simulink model "sys"  (R2025b)
settings: Solver=FixedStepDiscrete  StartTime=0.0  StopTime=simin.Time.data(end)  FixedStep=0.001  RelTol=1e-3
model workspace (MAT data in the model file):
  Fz_stat_FL = Simulink.Parameter
  Fz_stat_FL.Value = 3921.3656
  Fz_stat_FL.Complexity = 'real'
  Fz_stat_FL.Dimensions = [1 1]
  Fz_stat_FL.DataType = 'double'
  Fz_stat_FL.DocUnits = 'N'
  Fz_stat_FR = Simulink.Parameter
  Fz_stat_FR.Value = 3921.3656
  Fz_stat_FR.Complexity = 'real'
  Fz_stat_FR.Dimensions = [1 1]
  Fz_stat_FR.DataType = 'double'
  Fz_stat_FR.DocUnits = 'N'
  Fz_stat_RL = Simulink.Parameter
  Fz_stat_RL.Value = 3922.1269
  Fz_stat_RL.Complexity = 'real'
  Fz_stat_RL.Dimensions = [1 1]
  Fz_stat_RL.DataType = 'double'
  Fz_stat_RL.DocUnits = 'N'
  Fz_stat_RR = Simulink.Parameter
  Fz_stat_RR.Value = 3922.1267
  Fz_stat_RR.Complexity = 'real'
  Fz_stat_RR.Dimensions = [1 1]
  Fz_stat_RR.DataType = 'double'
  Fz_stat_RR.DocUnits = 'N'
  cog_height = Simulink.Parameter
  cog_height.Value = 0.604
  cog_height.Complexity = 'real'
  cog_height.Dimensions = [1 1]
  cog_height.DataType = 'double'
  cog_height.DocUnits = 'm'
  g = Simulink.Parameter
  g.Value = 9.806
  g.Complexity = 'real'
  g.Dimensions = [1 1]
  g.DataType = 'double'
  g.DocUnits = 'm/s^2'
  lF = Simulink.Parameter
  lF.Value = 1.466
  lF.Complexity = 'real'
  lF.Dimensions = [1 1]
  lF.DataType = 'double'
  lF.DocUnits = 'm'
  lR = Simulink.Parameter
  lR.Value = 1.509
  lR.Complexity = 'real'
  lR.Dimensions = [1 1]
  lR.DataType = 'double'
  lR.DocUnits = 'm'
  pitchAngle = Simulink.Parameter
  pitchAngle.Value = [0.00443372596055 0.00472012698538 0.00500652801021 0.00529292903504 0.00557933005986 0.00586573108469 0.00615213210952 0.00643853313435 0.00672493415917 0.007011335184 0.00729773620883 0.00758413723366 ... (200 elements, 200x1)]
  pitchAngle.Complexity = 'real'
  pitchAngle.Dimensions = [200 1]
  pitchAngle.DataType = 'double'
  pitchAngle.DocUnits = 'rad'
  pitchStiffness = Simulink.Parameter
  pitchStiffness.Value = [286621.759635 286644.842257 286407.773968 286374.136656 286600.567598 286901.705993 287109.32323 287190.659823 287245.018359 287344.728913 287488.533524 287631.863692 ... (200 elements, 200x1)]
  pitchStiffness.Complexity = 'real'
  pitchStiffness.Dimensions = [200 1]
  pitchStiffness.DataType = 'double'
  pitchStiffness.DocUnits = 'N*m/rad'
  pitch_inertia = Simulink.Parameter
  pitch_inertia.Value = 2180.5
  pitch_inertia.Complexity = 'real'
  pitch_inertia.Dimensions = [1 1]
  pitch_inertia.DataType = 'double'
  pitch_inertia.DocUnits = 'kg * m^2'
  pitching_coefficient = Simulink.Parameter
  pitching_coefficient.Value = -0.002
  pitching_coefficient.Complexity = 'real'
  pitching_coefficient.Dimensions = [1 1]
  pitching_coefficient.DataType = 'double'
  pitching_coefficient.DocUnits = '1'
  r = 0.9402
  rdyn = Simulink.Parameter
  rdyn.Value = 0.309
  rdyn.Complexity = 'real'
  rdyn.Dimensions = [1 1]
  rdyn.DataType = 'double'
  rdyn.DocUnits = 'm'
  reference_area = Simulink.Parameter
  reference_area.Value = 2.4
  reference_area.Complexity = 'real'
  reference_area.Dimensions = [1 1]
  reference_area.DataType = 'double'
  reference_area.DocUnits = 'kg / m^3'
  rho = Simulink.Parameter
  rho.Value = 1.2
  rho.Complexity = 'real'
  rho.Dimensions = [1 1]
  rho.DataType = 'double'
  rho.DocUnits = 'm^2'
  rollStiffness_F = Simulink.Parameter
  rollStiffness_F.Value = -66168.4036
  rollStiffness_F.Complexity = 'real'
  rollStiffness_F.Dimensions = [1 1]
  rollStiffness_F.DataType = 'double'
  rollStiffness_F.DocUnits = 'N*m/rad'
  rollStiffness_R = Simulink.Parameter
  rollStiffness_R.Value = -79058.3706
  rollStiffness_R.Complexity = 'real'
  rollStiffness_R.Dimensions = [1 1]
  rollStiffness_R.DataType = 'double'
  rollStiffness_R.DocUnits = 'N*m/rad'
  sprung_mass = Simulink.Parameter
  sprung_mass.Value = 1373.3
  sprung_mass.Complexity = 'real'
  sprung_mass.Dimensions = [1 1]
  sprung_mass.DataType = 'double'
  sprung_mass.DocUnits = 'kg'
  total_pitchDamping = Simulink.Parameter
  total_pitchDamping.Value = 22000
  total_pitchDamping.Complexity = 'real'
  total_pitchDamping.Dimensions = [1 1]
  total_pitchDamping.DataType = 'double'
  total_pitchDamping.DocUnits = 'N*m/rad'
  total_pitchStiffness = Simulink.Parameter
  total_pitchStiffness.Value = 291158.1055
  total_pitchStiffness.Complexity = 'real'
  total_pitchStiffness.Dimensions = [1 1]
  total_pitchStiffness.DataType = 'double'
  total_pitchStiffness.DocUnits = 'N*m/rad'
  total_rollStiffness = Simulink.Parameter
  total_rollStiffness.Value = 138201.9734
  total_rollStiffness.Complexity = 'real'
  total_rollStiffness.Dimensions = [1 1]
  total_rollStiffness.DataType = 'double'
  total_rollStiffness.DocUnits = 'N*m/rad'
  total_rollStifness = Simulink.Parameter
  total_rollStifness.Value = 138201.9734
  total_rollStifness.Complexity = 'real'
  total_rollStifness.Dimensions = [1 1]
  total_rollStifness.DataType = 'double'
  total_rollStifness.DocUnits = 'Nm/rad'
  trackwidth_F = Simulink.Parameter
  trackwidth_F.Value = 1.6
  trackwidth_F.Complexity = 'real'
  trackwidth_F.Dimensions = [1 1]
  trackwidth_F.DataType = 'double'
  trackwidth_F.DocUnits = 'm'
  trackwidth_R = Simulink.Parameter
  trackwidth_R.Value = 1.614
  trackwidth_R.Complexity = 'real'
  trackwidth_R.Dimensions = [1 1]
  trackwidth_R.DataType = 'double'
  trackwidth_R.DocUnits = 'm'
  unsprung_mass = Simulink.Parameter
  unsprung_mass.Value = 226.704
  unsprung_mass.Complexity = 'real'
  unsprung_mass.Dimensions = [1 1]
  unsprung_mass.DataType = 'double'
  unsprung_mass.DocUnits = 'kg'
  wheelbase = Simulink.Parameter
  wheelbase.Value = 2.975
  wheelbase.Complexity = 'real'
  wheelbase.Dimensions = [1 1]
  wheelbase.DataType = 'double'
  wheelbase.DocUnits = 'm'
undefined symbols (not defined in the file): DiscIntNeverNeededParam
settings Model: Creator=I012488  LastModifiedBy=marcelkaminski
settings DebuggingCC: UnconnectedInputMsg=warning  UnconnectedOutputMsg=warning  UnconnectedLineMsg=warning
settings ModelReferenceCC: EnableRefExpFcnMdlSchedulingChecks=on
settings RTWCC: GPUComputeCapability=3.5  DLArmComputeVersion=19.05

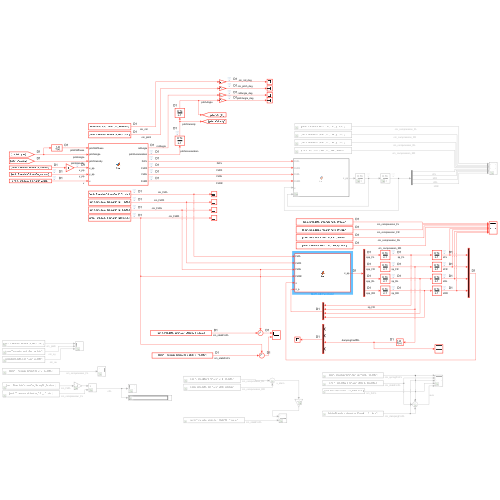
[thumbnail: Simulink's stored preview of the top-level diagram]
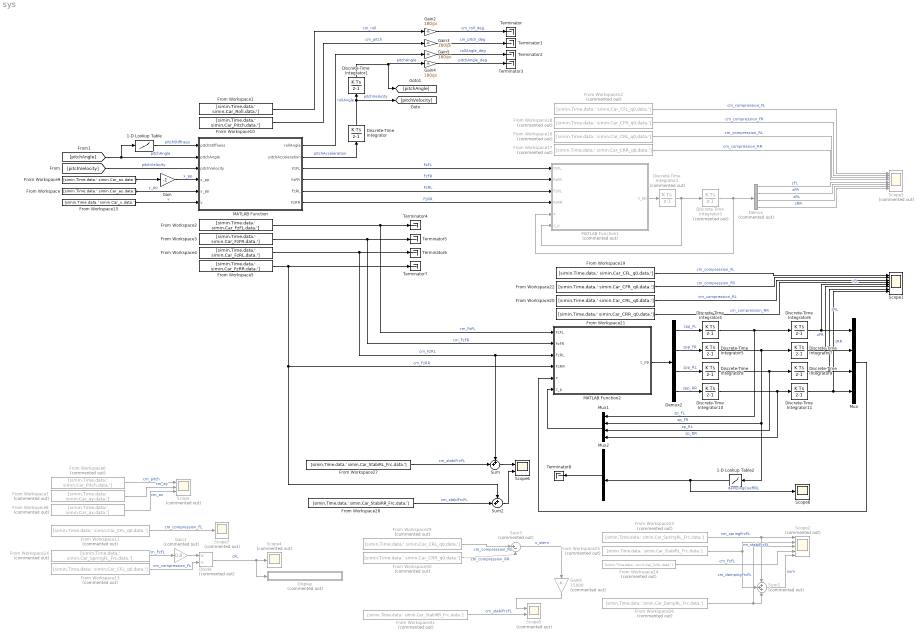
== system sys ==
  1-D Lookup Table : Lookup_n-D  NumberOfTableDimensions=1  BreakpointsForDimension1=pitchAngle  Table=pitchStiffness  InternalRulePriority=Speed  RndMeth=Simplest
  1-D Lookup Table2 : Lookup_n-D  NumberOfTableDimensions=1  BreakpointsForDimension1=[-1 -0.1 0 0.1 1]  Table="[2055.90  31.359 0 18.453 756.31]"  InternalRulePriority=Speed  RndMeth=Simplest
  Demux : Demux  Commented=on
  Demux2 : Demux
  Discrete-Time Integrator{,4..8,10..11} (8 alike) : DiscreteIntegrator  SampleTime=-1  ICPrevOutput=DiscIntNeverNeededParam  ICPrevScaledInput=DiscIntNeverNeededParam
  Discrete-Time Integrator1 : DiscreteIntegrator  InitialCondition=-0.001  SampleTime=-1  ICPrevOutput=DiscIntNeverNeededParam  ICPrevScaledInput=DiscIntNeverNeededParam
  Discrete-Time Integrator2 : DiscreteIntegrator  Commented=on  SampleTime=-1  ICPrevOutput=DiscIntNeverNeededParam  ICPrevScaledInput=DiscIntNeverNeededParam
  Discrete-Time Integrator3 : DiscreteIntegrator  Commented=on  SampleTime=-1  ICPrevOutput=DiscIntNeverNeededParam  ICPrevScaledInput=DiscIntNeverNeededParam
  Discrete-Time Integrator9 : DiscreteIntegrator  InitialCondition=-0.0007  SampleTime=-1  ICPrevOutput=DiscIntNeverNeededParam  ICPrevScaledInput=DiscIntNeverNeededParam
  Display : Display  Commented=on
      settings: Format=long_e
  Divide : Product  Commented=on  Inputs=*/
  From Workspace : FromWorkspace  VariableName=[simin.Time.data.' simin.Car_ay.data.']  SampleTime=0.01
  From Workspace1 : FromWorkspace  VariableName=[simin.Time.data.' simin.Car_Roll.data.']  SampleTime=0.01
  From Workspace10 : FromWorkspace  VariableName=[simin.Time.data.' simin.Car_Pitch.data.']  SampleTime=0.01
  From Workspace11 : FromWorkspace  Commented=on  VariableName=[simin.Time.data.' simin.Car_CFL_q0.data.']
  From Workspace12 : FromWorkspace  Commented=on  VariableName=[simin.Time.data.' simin.Car_CFL_q0.data.']  SampleTime=0.01
  From Workspace13 : FromWorkspace  Commented=on  VariableName=[simin.Time.data.' simin.Car_CFL_q0.data.']
  From Workspace14 : FromWorkspace  Commented=on  VariableName=[simin.Time.data.' simin.Car_SpringFL_Frc.data.']
  From Workspace15 : FromWorkspace  VariableName=[simin.Time.data.' simin.Car_v.data.']  SampleTime=0.01
  From Workspace16 : FromWorkspace  Commented=on  VariableName=[simin.Time.data.' simin.Car_CRL_q0.data.']  SampleTime=0.01
  From Workspace17 : FromWorkspace  Commented=on  VariableName=[simin.Time.data.' simin.Car_CRR_q0.data.']  SampleTime=0.01
  From Workspace18 : FromWorkspace  Commented=on  VariableName=[simin.Time.data.' simin.Car_CFR_q0.data.']  SampleTime=0.01
  From Workspace19 : FromWorkspace  VariableName=[simin.Time.data.' simin.Car_CFL_q0.data.']  SampleTime=0.01
  From Workspace2 : FromWorkspace  VariableName=[simin.Time.data.' simin.Car_FzFL.data.']  SampleTime=0.01
  From Workspace20 : FromWorkspace  VariableName=[simin.Time.data.' simin.Car_CRL_q0.data.']  SampleTime=0.01
  From Workspace21 : FromWorkspace  VariableName=[simin.Time.data.' simin.Car_CRR_q0.data.']  SampleTime=0.01
  From Workspace22 : FromWorkspace  VariableName=[simin.Time.data.' simin.Car_CFR_q0.data.']  SampleTime=0.01
  From Workspace23 : FromWorkspace  Commented=on  VariableName=[simin.Time.data.' simin.Car_SpringRL_Frc.data.']  SampleTime=0.01
  From Workspace24 : FromWorkspace  Commented=on  VariableName=[simin.Time.data.' simin.Car_FzRL.data.']  SampleTime=0.01
  From Workspace25 : FromWorkspace  Commented=on  VariableName=[simin.Time.data.' simin.Car_StabiRL_Frc.data.']  SampleTime=0.01
  From Workspace26 : FromWorkspace  Commented=on  VariableName=[simin.Time.data.' simin.Car_DampRL_Frc.data.']  SampleTime=0.01
  From Workspace27 : FromWorkspace  VariableName=[simin.Time.data.' simin.Car_StabiRL_Frc.data.']  SampleTime=0.01
  From Workspace28 : FromWorkspace  VariableName=[simin.Time.data.' simin.Car_StabiRR_Frc.data.']  SampleTime=0.01
  From Workspace29 : FromWorkspace  Commented=on  VariableName=[simin.Time.data.' simin.Car_CRL_q0.data.']  SampleTime=0.01
  From Workspace3 : FromWorkspace  VariableName=[simin.Time.data.' simin.Car_FzFR.data.']  SampleTime=0.01
  From Workspace30 : FromWorkspace  Commented=on  VariableName=[simin.Time.data.' simin.Car_CRR_q0.data.']  SampleTime=0.01
  From Workspace31 : FromWorkspace  Commented=on  VariableName=[simin.Time.data.' simin.Car_StabiRR_Frc.data.']  SampleTime=0.01
  From Workspace4 : FromWorkspace  VariableName=[simin.Time.data.' simin.Car_FzRL.data.']  SampleTime=0.01
  From Workspace5 : FromWorkspace  VariableName=[simin.Time.data.' simin.Car_FzRR.data.']  SampleTime=0.01
  From Workspace6 : FromWorkspace  Commented=on  VariableName=[simin.Time.data.' simin.Car_Pitch.data.']
  From Workspace7 : FromWorkspace  Commented=on  VariableName=[simin.Time.data.' simin.Car_ay.data.']
  From Workspace8 : FromWorkspace  Commented=on  VariableName=[simin.Time.data.' simin.Car_ax.data.']
  From Workspace9 : FromWorkspace  VariableName=[simin.Time.data.' simin.Car_ax.data.']  SampleTime=0.01
  Gain : Gain  Gain=-1
  Gain1 : Gain  Commented=on  Gain=0.8
  Gain{2..5} (4 alike) : Gain  Gain=180/pi
  Gain6 : Gain  Commented=on  Gain=15000
  MATLAB Function : MATLAB Function  TreatAsAtomicUnit=on
  MATLAB Function1 : MATLAB Function  Commented=on  TreatAsAtomicUnit=on
  MATLAB Function2 : MATLAB Function  TreatAsAtomicUnit=on
  Mux : Mux
  Mux1 : Mux
  Mux2 : Mux
  Scope : Scope  Commented=on  NumInputPorts=3
      settings: ActiveDisplayYMinimum=-0.00699  ActiveDisplayYMaximum=0.02856  DataLoggingVariableName=ScopeData2
  Scope1 : Scope  NumInputPorts=8
      settings: ActiveDisplayYMinimum=-0.057258109748267769  ActiveDisplayYMaximum=0.059973873910534263
  Scope2 : Scope  Commented=on  NumInputPorts=5
      settings: ActiveDisplayYMinimum=-519.06918168067921  ActiveDisplayYMaximum=4484.9822962284088  DataLoggingVariableName=ScopeData4
  Scope3 : Scope  Commented=on  NumInputPorts=8
      settings: ActiveDisplayYMinimum=-0.094623233695607184  ActiveDisplayYMaximum=0.027480534772711229  DataLoggingVariableName=ScopeData2
  Scope4 : Scope  Commented=on
      settings: ActiveDisplayYMinimum=-6.64271465116E+8  ActiveDisplayYMaximum=3.41636027705721E+9  DataLoggingVariableName=ScopeData3
  Scope5 : Scope  Commented=on  NumInputPorts=2
      settings: ActiveDisplayYMinimum=-982.79968407035688  ActiveDisplayYMaximum=303.75455820689251  DataLoggingVariableName=ScopeData5
  Scope6 : Scope  NumInputPorts=2
      settings: ActiveDisplayYMinimum=-1  ActiveDisplayYMaximum=1  DataLoggingVariableName=ScopeData6
  Scope7 : Scope  Commented=on
      settings: ActiveDisplayYMinimum=-0.02942  ActiveDisplayYMaximum=0.01092
  Scope8 : Scope
      settings: ActiveDisplayYMinimum=-0.83271159099636516  ActiveDisplayYMaximum=7.4944043189672884  DataLoggingVariableName=ScopeData7
  Sum : Sum  Inputs=++|
  Sum1 : Sum  Commented=on  Inputs=+++
  Sum2 : Sum  Inputs=++|
  Sum3 : Sum  Commented=on  Inputs=|+-
  Terminator{,1..8} (9 alike) : Terminator
  wires:
  MATLAB Function/3(FzFL) -> MATLAB Function1/1(FzFL)  "FzFL"
  From Workspace/1 -> MATLAB Function/5(y_pp)  "y_pp"
  MATLAB Function/1(rollAngle) -> Gain5/1  "rollAngle"
  From Workspace1/1 -> Gain2/1  "cm_roll"
  From Workspace2/1 -> MATLAB Function2/1(FzFL), Terminator4/1  "cm_FzFL"
  MATLAB Function/4(FzFR) -> MATLAB Function1/2(FzFR)  "FzFR"
  MATLAB Function/5(FzRL) -> MATLAB Function1/3(FzRL)  "FzRL"
  MATLAB Function/6(FzRR) -> MATLAB Function1/4(FzRR)  "FzRR"
  From Workspace3/1 -> MATLAB Function2/2(FzFR), Terminator5/1  "cm_FzFR"
  From Workspace4/1 -> Sum/1, MATLAB Function2/3(FzRL), Terminator6/1  "cm_FzRL"
  From Workspace5/1 -> Terminator7/1, Sum2/1, MATLAB Function2/4(FzRR)  "cm_FzRR"
  From Workspace6/1 -> Scope/1  "cm_pitch"
  From Workspace7/1 -> Scope/2  "cm_ay"
  From Workspace8/1 -> Scope/3  "cm_ax"
  From Workspace9/1 -> Gain/1
  MATLAB Function1/1(z_pp) -> Discrete-Time Integrator2/1
  MATLAB Function/2(pitchAcceleration) -> Discrete-Time Integrator/1  "pitchAcceleration"
  From Workspace10/1 -> Gain3/1  "cm_pitch"
  Gain/1 -> MATLAB Function/4(x_pp)  "x_pp"
  From Workspace11/1 -> Scope7/1  "cm_compression_FL"
  From Workspace12/1 -> Scope3/1  "cm_compression_FL"
  Discrete-Time Integrator2/1 -> MATLAB Function1/6(z_p), Discrete-Time Integrator3/1
  Discrete-Time Integrator3/1 -> MATLAB Function1/5(z), Demux/1
  From Workspace14/1 -> Gain1/1  "cm_FzFL"
  From Workspace13/1 -> Divide/2  "cm_compression_FL"
  Divide/1 -> Display/1, Scope4/1  "cFL"
  Gain1/1 -> Divide/1
  Discrete-Time Integrator/1 -> [pitchVelocity], Discrete-Time Integrator1/1  "pitchVelocity"
  Discrete-Time Integrator1/1 -> Gain4/1, [pitchAngle]  "pitchAngle"
  [pitchVelocity] -> MATLAB Function/3(pitchVelocity)  "pitchVelocity"
  [pitchAngle] -> 1-D Lookup Table/1, MATLAB Function/2(pitchAngle)  "pitchAngle"
  From Workspace15/1 -> MATLAB Function/6(v)  "v"
  1-D Lookup Table/1 -> MATLAB Function/1(pitchStiffness)  "pitchStiffness"
  Gain2/1 -> Terminator/1  "cm_roll_deg"
  Gain3/1 -> Terminator1/1  "cm_pitch_deg"
  Gain4/1 -> Terminator3/1  "pitchAngle_deg"
  Gain5/1 -> Terminator2/1  "rollAngle_deg"
  From Workspace18/1 -> Scope3/2  "cm_compression_FR"
  From Workspace16/1 -> Scope3/3  "cm_compression_RL"
  From Workspace17/1 -> Scope3/4  "cm_compression_RR"
  Demux/1 -> Scope3/5  "zFL"
  Demux/2 -> Scope3/6  "zFR"
  Demux/3 -> Scope3/7  "zRL"
  Demux/4 -> Scope3/8  "zRR"
  From Workspace22/1 -> Scope1/2  "cm_compression_FR"
  From Workspace21/1 -> Scope1/4  "cm_compression_RR"
  From Workspace20/1 -> Scope1/3  "cm_compression_RL"
  MATLAB Function2/1(z_pp) -> Demux2/1
  From Workspace19/1 -> Scope1/1  "cm_compression_FL"
  Mux/1 -> MATLAB Function2/5(z)
  From Workspace23/1 -> Scope2/1, Sum1/1  "cm_springFrcFL"
  From Workspace24/1 -> Scope2/4  "cm_FzFL"
  From Workspace25/1 -> Scope2/2, Sum1/2  "cm_stabiFrcFL"
  Sum1/1 -> Scope2/5  "sum"
  From Workspace26/1 -> Scope2/3, Sum1/3  "cm_dampingFrcFL"
  From Workspace27/1 -> Sum/2  "cm_stabiFrcFL"
  Sum/1 -> Scope6/1
  From Workspace28/1 -> Sum2/2  "cm_stabiFrcFL"
  Sum2/1 -> Scope6/2
  From Workspace29/1 -> Sum3/1  "cm_compression_RL"
  From Workspace30/1 -> Sum3/2  "cm_compression_RR"
  Sum3/1 -> Gain6/1  "x_stern"
  Gain6/1 -> Scope5/1
  From Workspace31/1 -> Scope5/2  "cm_stabiFrcFL"
  Demux2/1 -> Discrete-Time Integrator4/1  "zpp_FL"
  Discrete-Time Integrator4/1 -> Mux1/1, Discrete-Time Integrator6/1  "zp_FL"
  Discrete-Time Integrator6/1 -> Mux/1, Scope1/5  "zFL"
  Discrete-Time Integrator7/1 -> Mux/2, Scope1/6  "zFR"
  Discrete-Time Integrator5/1 -> Mux1/2, 1-D Lookup Table2/1, Discrete-Time Integrator7/1  "zp_FR"
  Demux2/2 -> Discrete-Time Integrator5/1  "zpp_FR"
  Demux2/3 -> Discrete-Time Integrator8/1  "zpp_RL"
  Discrete-Time Integrator8/1 -> Mux1/3, Discrete-Time Integrator9/1  "zp_RL"
  Discrete-Time Integrator9/1 -> Scope1/7, Mux/3  "zRL"
  Demux2/4 -> Discrete-Time Integrator10/1  "zpp_RR"
  Discrete-Time Integrator10/1 -> Mux1/4, Discrete-Time Integrator11/1  "zp_RR"
  Discrete-Time Integrator11/1 -> Scope1/8, Mux/4  "zRR"
  Mux1/1 -> MATLAB Function2/6(z_p)
  1-D Lookup Table2/1 -> Scope8/1, Mux2/3  "dampingCoeffRL"
  Mux2/1 -> Terminator8/1

== matlab function sys/MATLAB Function2 ==
  data: FzFL input; z_pp output; FzFR input; FzRL input; FzRR input; z input size=[4 1]; z_p input size=[4 1]; Fz_stat_FL parameter; Fz_stat_FR parameter; Fz_stat_RL parameter; Fz_stat_RR parameter
function z_pp = fcn(FzFL,FzFR,FzRL,FzRR,z,z_p,Fz_stat_FL,Fz_stat_FR,Fz_stat_RL,Fz_stat_RR)
g = 9.806;

cFL = 9.976e+04;  bFL = 2179;
cFR = 35000.0;  bFR = 2179.0;
cRL = 40000; % bRL = 2179.0;
cRR = 40000;  bRR = 2179.0;

c_anti_roll_R = 15000;

mFL = Fz_stat_FL ./ g;
mFR = Fz_stat_FR ./ g;
mRL = Fz_stat_RL ./ g;
mRR = Fz_stat_RR ./ g;

z_p_FL = z_p(1);
z_p_FR = z_p(2);
z_p_RL = z_p(3);
z_p_RR = z_p(4);

bRL = 2500;
if z_p_RL <= 0
    bRL = 2500;
elseif z_p_RL > 0
    bRL = 5000;
end

z_FL = z(1);
z_FR = z(2);
z_RL = z(3);
z_RR = z(4);

anti_rollbar_frc_R = c_anti_roll_R .* (z_RR - z_RL);

z_pp_FL = (FzFL - bFL .* z_p_FL - cFL .* z_FL) ./ mFL - g;
z_pp_FR = (FzFR - bFR .* z_p_FR - cFR .* z_FR) ./ mFR - g;
z_pp_RL = (FzRL - bRL .* z_p_RL - cRL .* z_RL + anti_rollbar_frc_R) ./ mRL - g;
z_pp_RR = (FzRR - bRR .* z_p_RR - cRR .* z_RR - anti_rollbar_frc_R) ./ mRR - g;

z_pp = zeros(4,1);
z_pp(1) = z_pp_FL;
z_pp(2) = z_pp_FR;
z_pp(3) = z_pp_RL;
z_pp(4) = z_pp_RR;

== matlab function sys/MATLAB Function1 ==
  data: FzFL input; z_pp output; FzFR input; FzRL input; FzRR input; z input size=[4 1]; z_p input size=[4 1]; Fz_stat_FL parameter; Fz_stat_FR parameter; Fz_stat_RL parameter; Fz_stat_RR parameter
function z_pp = fcn(FzFL,FzFR,FzRL,FzRR,z,z_p,Fz_stat_FL,Fz_stat_FR,Fz_stat_RL,Fz_stat_RR)
g = 9.806;

cFL = 9.976e+04;  bFL = 2179;
cFR = 35000.0;  bFR = 2179.0;
cRL = 1.77*40000.0;  bRL = 2179.0;
cRR = 1.77*40000.0;  bRR = 2179.0;

mFL = Fz_stat_FL ./ g;
mFR = Fz_stat_FR ./ g;
mRL = Fz_stat_RL ./ g;
mRR = Fz_stat_RR ./ g;

z_p_FL = z_p(1);
z_p_FR = z_p(2);
z_p_RL = z_p(3);
z_p_RR = z_p(4);

z_FL = z(1);
z_FR = z(2);
z_RL = z(3);
z_RR = z(4);

z_pp_FL = (FzFL - bFL .* z_p_FL - cFL .* z_FL) ./ mFL - g;
z_pp_FR = (FzFR - bFR .* z_p_FR - cFR .* z_FR) ./ mFR - g;
z_pp_RL = (FzRL - bRL .* z_p_RL - cRL .* z_RL) ./ mRL - g;
z_pp_RR = (FzRR - bRR .* z_p_RR - cRR .* z_RR) ./ mRR - g;

z_pp = zeros(4,1);
z_pp(1) = z_pp_FL;
z_pp(2) = z_pp_FR;
z_pp(3) = z_pp_RL;
z_pp(4) = z_pp_RR;

== matlab function sys/MATLAB Function ==
  data: pitchStiffness input; pitchAngle input; pitchVelocity input; x_pp input; rollAngle output; pitchAcceleration output; y_pp input; v input; cog_height parameter; sprung_mass parameter; FzFL output; rollStiffness_F parameter; rollStiffness_R parameter; total_rollStiffness parameter; trackwidth_F parameter; trackwidth_R parameter; Fz_stat_FL parameter; Fz_stat_FR parameter; Fz_stat_RL parameter; Fz_stat_RR parameter; FzFR output; FzRL output; FzRR output; wheelbase parameter; total_pitchStiffness parameter; rdyn parameter; unsprung_mass parameter; pitch_inertia parameter; total_pitchDamping parameter; reference_area parameter; pitching_coefficient parameter; rho parameter
function [rollAngle,pitchAcceleration,FzFL,FzFR,FzRL,FzRR]  = fcn(pitchStiffness,pitchAngle,pitchVelocity,x_pp, y_pp,v, cog_height, sprung_mass,rollStiffness_F,rollStiffness_R,total_rollStiffness,trackwidth_F, trackwidth_R, Fz_stat_FL, Fz_stat_FR, Fz_stat_RL, Fz_stat_RR, wheelbase, total_pitchStiffness, rdyn, unsprung_mass, pitch_inertia, total_pitchDamping, reference_area, pitching_coefficient, rho)

rollTorque = sprung_mass .* y_pp .* cog_height;
rollAngle = rollTorque ./ (total_rollStiffness);

dFz_roll_FL = (rollAngle .* rollStiffness_F - rdyn .* unsprung_mass .* y_pp) ./ trackwidth_F;
dFz_roll_FR = (rollAngle .* rollStiffness_F - rdyn .* unsprung_mass .* y_pp) ./ trackwidth_F;
dFz_roll_RL = (rollAngle .* rollStiffness_R - rdyn .* unsprung_mass .* y_pp) ./ trackwidth_R;
dFz_roll_RR = (rollAngle .* rollStiffness_R - rdyn .* unsprung_mass .* y_pp) ./ trackwidth_R;
           
pitchTorque = sprung_mass .* x_pp .* cog_height - rho ./2 .* pitching_coefficient .* wheelbase .* reference_area .* v^2;
% pitchStiffness = 3.825903e+09 * pitchAngle^3 + -1.854731e+09 * pitchAngle^2 + 1.728035e+08 * pitchAngle + -1.759672e+06;
% pitchStiffness = min(max(pitchStiffness, 290e3), 626e3);
pitchAcceleration = (pitchTorque - total_pitchDamping .* pitchVelocity - pitchStiffness .* pitchAngle) ./ pitch_inertia;

dFz_pitch_FL = (pitchStiffness ./ 2 .* pitchAngle + total_pitchDamping ./ 2 .* pitchVelocity - pitch_inertia ./4 .* pitchAcceleration) ./ wheelbase;
dFz_pitch_FR = (pitchStiffness ./ 2 .* pitchAngle + total_pitchDamping ./ 2 .* pitchVelocity - pitch_inertia ./4 .* pitchAcceleration) ./ wheelbase;
dFz_pitch_RL = (pitchStiffness ./ 2 .* pitchAngle + total_pitchDamping ./ 2 .* pitchVelocity - pitch_inertia ./4 .* pitchAcceleration) ./ wheelbase;
dFz_pitch_RR = (pitchStiffness ./ 2 .* pitchAngle + total_pitchDamping ./ 2 .* pitchVelocity - pitch_inertia ./4 .* pitchAcceleration) ./ wheelbase;

FzFL = Fz_stat_FL + dFz_roll_FL + dFz_pitch_FL;
FzFR = Fz_stat_FR - dFz_roll_FR + dFz_pitch_FR;
FzRL = Fz_stat_RL + dFz_roll_RL - dFz_pitch_RL;
FzRR = Fz_stat_RR - dFz_roll_RR - dFz_pitch_RR;
